simulink model "FixedWing_Dynamic_Model_SIL_PX4"  (R2022b)
settings: Solver=ode4  StartTime=0.0  StopTime=inf  FixedStep=0.004  RelTol=1e-3
model workspace (MAT data in the model file):
  sample_time = 0.004
values from neighbouring files (symbols this model uses):
  uavData = struct    [InitFixedWingParam.m]
undefined symbols (not defined in the file or in its folder): Earth, env, WGS84
libraries: aerolibactuator x5, simulink_extras x3, aerolibasang x2, aerolibatmos2 x2, shared6dof x1, aerolibtransform2 x1, aerolibconvert2 x1, aerolibanimutils x1
(part 2 of 2)

== system FixedWing_Dynamic_Model_SIL_PX4/Fixed-wing UAV Dynamics/Force and Moment Calculation/Aerodynamic Forces and Moments/Compute Body Frame Forces and Moments/Rotate FM to body frame/Rotate Moments/RB2W ==
  aoa beta : Inport
  11 : Fcn  Expr=u[3]*u[4]
  12 : Fcn  Expr=u[2]
  13 : Fcn  Expr=u[1]*u[4]
  21 : Fcn  Expr=-u[3]*u[2]
  22 : Fcn  Expr=u[4]
  23 : Fcn  Expr=-u[1]*u[2]
  31 : Fcn  Expr=-u[1]
  32 : Fcn  Expr=0
  33 : Fcn  Expr=u[3]
  Mux : Mux  Inputs=2
  Mux3 : Mux  Inputs=9
  Reshape 9x1->3x3 : Reshape  OutputDimensionality=Customize  OutputDimensions=[3,3]
  sincos : Trigonometry  Operator=sincos
  Rw2b : Outport  VectorParamsAs1DForOutWhenUnconnected=off
  wires:
  Mux/1 -> 11/1, 21/1, 31/1, 12/1, 22/1, 32/1, 13/1, 23/1, 33/1
  aoa beta/1 -> sincos/1
  sincos/2 -> Mux/2
  sincos/1 -> Mux/1
  33/1 -> Mux3/9
  23/1 -> Mux3/8
  13/1 -> Mux3/7
  32/1 -> Mux3/6
  22/1 -> Mux3/5
  12/1 -> Mux3/4
  31/1 -> Mux3/3
  21/1 -> Mux3/2
  11/1 -> Mux3/1
  Reshape 9x1->3x3/1 -> Rw2b/1
  Mux3/1 -> Reshape 9x1->3x3/1

== system FixedWing_Dynamic_Model_SIL_PX4/Fixed-wing UAV Dynamics/Force and Moment Calculation/Aerodynamic Forces and Moments/Compute Body Frame Forces and Moments/Wind frame F& M/Lateral Channel/CY ==
  beta : Inport
  dR : Inport  Port=2
  CYDr : Constant  Value=uavData.aero.CYDr
      settings: AttributesFormatString=%<Value>
  CYb : Constant  Value=uavData.aero.CYb
      settings: AttributesFormatString=%<Value>
  Product : Product  SaturateOnIntegerOverflow=on  OutDataTypeStr=Inherit: Same as first input
  Product1 : Product  SaturateOnIntegerOverflow=on  OutDataTypeStr=Inherit: Same as first input
  Sum2 : Sum  SaturateOnIntegerOverflow=on
  CY : Outport  VectorParamsAs1DForOutWhenUnconnected=off
  wires:
  Product1/1 -> Sum2/2
  dR/1 -> Product1/2
  CYDr/1 -> Product1/1
  Product/1 -> Sum2/1
  Sum2/1 -> CY/1
  beta/1 -> Product/2
  CYb/1 -> Product/1

== system FixedWing_Dynamic_Model_SIL_PX4/Fixed-wing UAV Dynamics/Force and Moment Calculation/Aerodynamic Forces and Moments/Compute Body Frame Forces and Moments/Wind frame F& M/Lateral Channel/Cl ==
  beta : Inport
  dA : Inport  Port=2
  dR : Inport  Port=3
  p,q,r : Inport  Port=4
  Airspeed : Inport  Port=5
  ClDa : Constant  Value=uavData.aero.ClDa
      settings: AttributesFormatString=%<Value>
  ClDr : Constant  Value=uavData.aero.ClDr
      settings: AttributesFormatString=%<Value>
  Clb : Constant  Value=uavData.aero.Clb
      settings: AttributesFormatString=%<Value>
  Product1 : Product  SaturateOnIntegerOverflow=on  OutDataTypeStr=Inherit: Same as first input
  Product4 : Product  SaturateOnIntegerOverflow=on  OutDataTypeStr=Inherit: Same as first input
  Product5 : Product  SaturateOnIntegerOverflow=on  OutDataTypeStr=Inherit: Same as first input
  Sum : Sum  Inputs=+++++  SaturateOnIntegerOverflow=on
  roll factors : Subsystem
  Cl : Outport  VectorParamsAs1DForOutWhenUnconnected=off
  wires:
  roll factors/1(Clp) -> Sum/4
  Product5/1 -> Sum/2  "CldA"
  Airspeed/1 -> roll factors/2(Airspeed)
  p,q,r/1 -> roll factors/1(p,q,r)
  roll factors/2(Clr) -> Sum/5
  Product1/1 -> Sum/3  "Cldr"
  Product4/1 -> Sum/1  "Clb"
  Sum/1 -> Cl/1
  dR/1 -> Product1/2
  ClDr/1 -> Product1/1
  dA/1 -> Product5/2
  ClDa/1 -> Product5/1
  beta/1 -> Product4/2
  Clb/1 -> Product4/1

== system FixedWing_Dynamic_Model_SIL_PX4/Fixed-wing UAV Dynamics/Force and Moment Calculation/Aerodynamic Forces and Moments/Compute Body Frame Forces and Moments/Wind frame F& M/Lateral Channel/Cn ==
  beta : Inport
  dA : Inport  Port=2
  Dr : Inport  Port=3
  p,q,r : Inport  Port=4
  Airspeed : Inport  Port=5
  CnDa : Constant  Value=uavData.aero.CnDa
      settings: AttributesFormatString=%<Value>
  CnDr : Constant  Value=uavData.aero.CnDr
      settings: AttributesFormatString=%<Value>
  Cnb : Constant  Value=uavData.aero.Cnb
      settings: AttributesFormatString=%<Value>
  Product1 : Product  SaturateOnIntegerOverflow=on  OutDataTypeStr=Inherit: Same as first input
  Product4 : Product  SaturateOnIntegerOverflow=on  OutDataTypeStr=Inherit: Same as first input
  Product5 : Product  SaturateOnIntegerOverflow=on  OutDataTypeStr=Inherit: Same as first input
  Sum : Sum  Inputs=+++++  SaturateOnIntegerOverflow=on
  yaw factors : Subsystem
  Cn : Outport  VectorParamsAs1DForOutWhenUnconnected=off
  wires:
  Airspeed/1 -> yaw factors/2(Airspeed)
  p,q,r/1 -> yaw factors/1(p,q,r)
  Cnb/1 -> Product4/1
  beta/1 -> Product4/2
  CnDa/1 -> Product5/1
  Product5/1 -> Sum/2
  dA/1 -> Product5/2
  CnDr/1 -> Product1/1
  Dr/1 -> Product1/2
  Sum/1 -> Cn/1
  Product1/1 -> Sum/3
  yaw factors/2(Cnr) -> Sum/5
  yaw factors/1(Cnp) -> Sum/4
  Product4/1 -> Sum/1

== system FixedWing_Dynamic_Model_SIL_PX4/Fixed-wing UAV Dynamics/Force and Moment Calculation/Aerodynamic Forces and Moments/Compute Body Frame Forces and Moments/Wind frame F& M/Longitudinal Channel/CD ==
  CL : Inport
  Apolar : Constant  Value=uavData.aero.A1
      settings: AttributesFormatString=%<Value>
  Apolar (A2) : Constant  Value=uavData.aero.Apolar
      settings: AttributesFormatString=%<Value>
  CD0 : Constant  Value=uavData.aero.CD0
      settings: AttributesFormatString=%<Value>
  Gain : Gain  Gain=-1  SaturateOnIntegerOverflow=on  OutDataTypeStr=Inherit: Same as input  ParamDataTypeStr=Inherit: Same as input
      settings: AttributesFormatString=%<Gain>
  Math Function : Math  Operator=square  SignedPower=on
  Product : Product  SaturateOnIntegerOverflow=on  OutDataTypeStr=Inherit: Same as first input
  Product1 : Product  SaturateOnIntegerOverflow=on  OutDataTypeStr=Inherit: Same as first input
  Sum1 : Sum  Inputs=+++  SaturateOnIntegerOverflow=on
  CD : Outport  VectorParamsAs1DForOutWhenUnconnected=off
  wires:
  Gain/1 -> CD/1
  Apolar (A2)/1 -> Product/1
  Math Function/1 -> Product/2
  Product1/1 -> Sum1/3
  Product/1 -> Sum1/2
  CL/1 -> Math Function/1, Product1/1
  Sum1/1 -> Gain/1
  CD0/1 -> Sum1/1
  Apolar/1 -> Product1/2

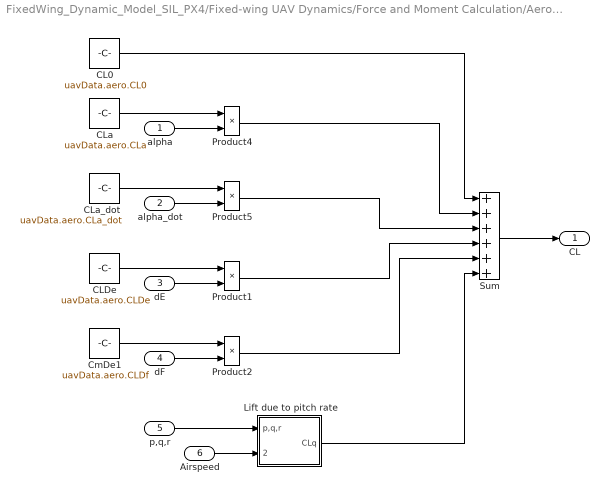
== system FixedWing_Dynamic_Model_SIL_PX4/Fixed-wing UAV Dynamics/Force and Moment Calculation/Aerodynamic Forces and Moments/Compute Body Frame Forces and Moments/Wind frame F& M/Longitudinal Channel/CL ==
  alpha : Inport
  alpha_dot : Inport  Port=2
  dE : Inport  Port=3
  dF : Inport  Port=4
  p,q,r : Inport  Port=5
  Airspeed : Inport  Port=6
  CL0 : Constant  Value=uavData.aero.CL0
      settings: AttributesFormatString=%<Value>
  CLDe : Constant  Value=uavData.aero.CLDe
      settings: AttributesFormatString=%<Value>
  CLa : Constant  Value=uavData.aero.CLa
      settings: AttributesFormatString=%<Value>
  CLa_dot : Constant  Value=uavData.aero.CLa_dot
      settings: AttributesFormatString=%<Value>
  CmDe1 : Constant  Value=uavData.aero.CLDf
      settings: AttributesFormatString=%<Value>
  Lift due to pitch rate : Subsystem
  Product{1..2,4..5} (4 alike) : Product  SaturateOnIntegerOverflow=on  OutDataTypeStr=Inherit: Same as first input
  Sum : Sum  Inputs=++++++  SaturateOnIntegerOverflow=on
  CL : Outport  VectorParamsAs1DForOutWhenUnconnected=off
  wires:
  CL0/1 -> Sum/1
  Airspeed/1 -> Lift due to pitch rate/2(Airspeed)
  p,q,r/1 -> Lift due to pitch rate/1(p,q,r)
  Lift due to pitch rate/1(CLq) -> Sum/6
  Product2/1 -> Sum/5
  Product1/1 -> Sum/4
  Product5/1 -> Sum/3
  CmDe1/1 -> Product2/1
  dF/1 -> Product2/2
  Sum/1 -> CL/1
  dE/1 -> Product1/2
  CLDe/1 -> Product1/1
  alpha_dot/1 -> Product5/2
  CLa_dot/1 -> Product5/1
  alpha/1 -> Product4/2
  CLa/1 -> Product4/1
  Product4/1 -> Sum/2

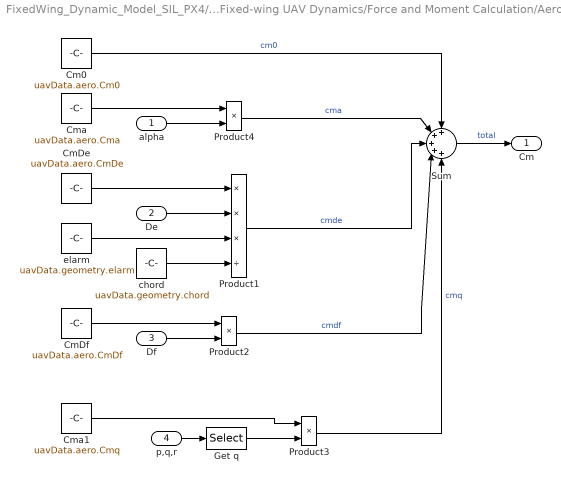
== system FixedWing_Dynamic_Model_SIL_PX4/Fixed-wing UAV Dynamics/Force and Moment Calculation/Aerodynamic Forces and Moments/Compute Body Frame Forces and Moments/Wind frame F& M/Longitudinal Channel/Cm ==
  alpha : Inport
  De : Inport  Port=2
  Df : Inport  Port=3
  p,q,r : Inport  Port=4
  Cm0 : Constant  Value=uavData.aero.Cm0
      settings: AttributesFormatString=%<Value>
  CmDe : Constant  Value=uavData.aero.CmDe
      settings: AttributesFormatString=%<Value>
  CmDf : Constant  Value=uavData.aero.CmDf
      settings: AttributesFormatString=%<Value>
  Cma : Constant  Value=uavData.aero.Cma
      settings: AttributesFormatString=%<Value>
  Cma1 : Constant  Value=uavData.aero.Cmq
      settings: AttributesFormatString=%<Value>
  Get q : Selector  InputPortWidth=3  IndexOptions=Index vector (dialog)  Indices=2  OutputSizes=[(-2)]
  Product1 : Product  Inputs=***/  SaturateOnIntegerOverflow=on  OutDataTypeStr=Inherit: Same as first input
  Product2 : Product  SaturateOnIntegerOverflow=on  OutDataTypeStr=Inherit: Same as first input
  Product3 : Product  SaturateOnIntegerOverflow=on  OutDataTypeStr=Inherit: Same as first input
  Product4 : Product  SaturateOnIntegerOverflow=on  OutDataTypeStr=Inherit: Same as first input
  Sum : Sum  Inputs=+++++  SaturateOnIntegerOverflow=on
  chord : Constant  Value=uavData.geometry.chord
      settings: AttributesFormatString=%<Value>
  elarm : Constant  Value=uavData.geometry.elarm
      settings: AttributesFormatString=%<Value>
  Cm : Outport  VectorParamsAs1DForOutWhenUnconnected=off
  wires:
  chord/1 -> Product1/4
  elarm/1 -> Product1/3
  Get q/1 -> Product3/2
  Product3/1 -> Sum/5  "cmq"
  p,q,r/1 -> Get q/1
  Cma1/1 -> Product3/1
  Product1/1 -> Sum/3  "cmde"
  Product4/1 -> Sum/2  "cma"
  Sum/1 -> Cm/1  "total"
  De/1 -> Product1/2
  CmDe/1 -> Product1/1
  alpha/1 -> Product4/2
  Cma/1 -> Product4/1
  Df/1 -> Product2/2
  CmDf/1 -> Product2/1
  Product2/1 -> Sum/4  "cmdf"
  Cm0/1 -> Sum/1  "cm0"

== system FixedWing_Dynamic_Model_SIL_PX4/Fixed-wing UAV Dynamics/Force and Moment Calculation/Aerodynamic Forces and Moments/Compute Body Frame Forces and Moments/Wind frame F& M/Lateral Channel/Cl/roll factors ==
  p,q,r : Inport
  Airspeed : Inport  Port=2
  Constant : Constant  Value=uavData.aero.Clp
      settings: AttributesFormatString=%<Value>
  Constant1 : Constant  Value=uavData.aero.Clr
      settings: AttributesFormatString=%<Value>
  Get p : Selector  InputPortWidth=3  IndexOptions=Index vector (dialog)  Indices=1  OutputSizes=[(-2)]
  Get r : Selector  InputPortWidth=3  IndexOptions=Index vector (dialog)  Indices=3  OutputSizes=[(-2)]
  Product : Product  SaturateOnIntegerOverflow=on  OutDataTypeStr=Inherit: Same as first input
  Product1 : Product  SaturateOnIntegerOverflow=on  OutDataTypeStr=Inherit: Same as first input
  roll rate fact : Subsystem
  yaw rate fact : Subsystem
  Clp : Outport  VectorParamsAs1DForOutWhenUnconnected=off
  Clr : Outport  Port=2  VectorParamsAs1DForOutWhenUnconnected=off
  wires:
  Get r/1 -> yaw rate fact/1(r)
  p,q,r/1 -> Get r/1, Get p/1
  Get p/1 -> roll rate fact/1(p)
  Airspeed/1 -> yaw rate fact/2(Airspeed), roll rate fact/2(Airspeed)
  yaw rate fact/1(Yaw Rate Fac) -> Product1/2
  Constant1/1 -> Product1/1
  roll rate fact/1(Roll Rate Fac) -> Product/2
  Constant/1 -> Product/1
  Product1/1 -> Clr/1
  Product/1 -> Clp/1

== system FixedWing_Dynamic_Model_SIL_PX4/Fixed-wing UAV Dynamics/Force and Moment Calculation/Aerodynamic Forces and Moments/Compute Body Frame Forces and Moments/Wind frame F& M/Lateral Channel/Cn/yaw factors ==
  p,q,r : Inport
  Airspeed : Inport  Port=2
  Constant : Constant  Value=uavData.aero.Cnp
      settings: AttributesFormatString=%<Value>
  Constant1 : Constant  Value=uavData.aero.Cnr
      settings: AttributesFormatString=%<Value>
  Get p : Selector  InputPortWidth=3  IndexOptions=Index vector (dialog)  Indices=1  OutputSizes=[(-2)]
  Get r : Selector  InputPortWidth=3  IndexOptions=Index vector (dialog)  Indices=3  OutputSizes=[(-2)]
  Product : Product  SaturateOnIntegerOverflow=on  OutDataTypeStr=Inherit: Same as first input
  Product1 : Product  SaturateOnIntegerOverflow=on  OutDataTypeStr=Inherit: Same as first input
  roll rate fact : Subsystem
  yaw rate fact : Subsystem
  Cnp : Outport  VectorParamsAs1DForOutWhenUnconnected=off
  Cnr : Outport  Port=2  VectorParamsAs1DForOutWhenUnconnected=off
  wires:
  Airspeed/1 -> yaw rate fact/2(Airspeed), roll rate fact/2(Airspeed)
  Get r/1 -> yaw rate fact/1(r)
  p,q,r/1 -> Get r/1, Get p/1
  Get p/1 -> roll rate fact/1(p)
  roll rate fact/1(Roll Rate Fac) -> Product/2
  Constant/1 -> Product/1
  yaw rate fact/1(Yaw Rate Fac) -> Product1/2
  Constant1/1 -> Product1/1
  Product1/1 -> Cnr/1
  Product/1 -> Cnp/1

== system FixedWing_Dynamic_Model_SIL_PX4/Fixed-wing UAV Dynamics/Force and Moment Calculation/Aerodynamic Forces and Moments/Compute Body Frame Forces and Moments/Wind frame F& M/Longitudinal Channel/CL/Lift due to pitch rate ==
  p,q,r : Inport
  Airspeed : Inport  Port=2
  Constant : Constant  Value=uavData.aero.CLq
      settings: AttributesFormatString=%<Value>
  Get q : Selector  InputPortWidth=3  IndexOptions=Index vector (dialog)  Indices=2  OutputSizes=[(-2)]
  Product : Product  SaturateOnIntegerOverflow=on  OutDataTypeStr=Inherit: Same as first input
  pitch rate factor : Subsystem
  CLq : Outport  VectorParamsAs1DForOutWhenUnconnected=off
  wires:
  Airspeed/1 -> pitch rate factor/2(Airspeed)
  Get q/1 -> pitch rate factor/1(q)
  p,q,r/1 -> Get q/1
  Product/1 -> CLq/1
  pitch rate factor/1(Pitch Rate Fac) -> Product/2
  Constant/1 -> Product/1

== system FixedWing_Dynamic_Model_SIL_PX4/Fixed-wing UAV Dynamics/Force and Moment Calculation/Aerodynamic Forces and Moments/Compute Body Frame Forces and Moments/Wind frame F& M/Lateral Channel/Cl/roll factors/roll rate fact ==
  p : Inport
  Airspeed : Inport  Port=2
  Cmq1 : Constant  Value=.5
      settings: AttributesFormatString=%<Value>
  Cmq2 : Constant  Value=uavData.geometry.span
      settings: AttributesFormatString=%<Value>
  Product : Product  Inputs=***/  SaturateOnIntegerOverflow=on  OutDataTypeStr=Inherit: Same as first input
  Saturation : Saturate  UpperLimit=inf  LowerLimit=0.1
      settings: AttributesFormatString="[%<LowerLimit>  %<UpperLimit>]"
  Roll Rate Fac : Outport  VectorParamsAs1DForOutWhenUnconnected=off
  wires:
  Saturation/1 -> Product/4
  Airspeed/1 -> Saturation/1
  Cmq2/1 -> Product/3
  Cmq1/1 -> Product/2
  p/1 -> Product/1
  Product/1 -> Roll Rate Fac/1

== system FixedWing_Dynamic_Model_SIL_PX4/Fixed-wing UAV Dynamics/Force and Moment Calculation/Aerodynamic Forces and Moments/Compute Body Frame Forces and Moments/Wind frame F& M/Lateral Channel/Cl/roll factors/yaw rate fact ==
  r : Inport
  Airspeed : Inport  Port=2
  Cmq3 : Constant  Value=.5
      settings: AttributesFormatString=%<Value>
  Cmq4 : Constant  Value=uavData.geometry.span
      settings: AttributesFormatString=%<Value>
  Product1 : Product  Inputs=***/  SaturateOnIntegerOverflow=on  OutDataTypeStr=Inherit: Same as first input
  Saturation : Saturate  UpperLimit=inf  LowerLimit=0.1
      settings: AttributesFormatString="[%<LowerLimit>  %<UpperLimit>]"
  Yaw Rate Fac : Outport  VectorParamsAs1DForOutWhenUnconnected=off
  wires:
  Product1/1 -> Yaw Rate Fac/1
  r/1 -> Product1/1
  Cmq3/1 -> Product1/2
  Cmq4/1 -> Product1/3
  Airspeed/1 -> Saturation/1
  Saturation/1 -> Product1/4

== system FixedWing_Dynamic_Model_SIL_PX4/Fixed-wing UAV Dynamics/Force and Moment Calculation/Aerodynamic Forces and Moments/Compute Body Frame Forces and Moments/Wind frame F& M/Lateral Channel/Cn/yaw factors/roll rate fact ==
  p : Inport
  Airspeed : Inport  Port=2
  Cmq1 : Constant  Value=.5
      settings: AttributesFormatString=%<Value>
  Cmq2 : Constant  Value=uavData.geometry.span
      settings: AttributesFormatString=%<Value>
  Product : Product  Inputs=***/  SaturateOnIntegerOverflow=on  OutDataTypeStr=Inherit: Same as first input
  Saturation : Saturate  UpperLimit=inf  LowerLimit=0.1
      settings: AttributesFormatString="[%<LowerLimit>  %<UpperLimit>]"
  Roll Rate Fac : Outport  VectorParamsAs1DForOutWhenUnconnected=off
  wires:
  Saturation/1 -> Product/4
  Airspeed/1 -> Saturation/1
  Cmq2/1 -> Product/3
  Cmq1/1 -> Product/2
  p/1 -> Product/1
  Product/1 -> Roll Rate Fac/1

== system FixedWing_Dynamic_Model_SIL_PX4/Fixed-wing UAV Dynamics/Force and Moment Calculation/Aerodynamic Forces and Moments/Compute Body Frame Forces and Moments/Wind frame F& M/Lateral Channel/Cn/yaw factors/yaw rate fact ==
  r : Inport
  Airspeed : Inport  Port=2
  Cmq3 : Constant  Value=.5
      settings: AttributesFormatString=%<Value>
  Cmq4 : Constant  Value=uavData.geometry.span
      settings: AttributesFormatString=%<Value>
  Product1 : Product  Inputs=***/  SaturateOnIntegerOverflow=on  OutDataTypeStr=Inherit: Same as first input
  Saturation : Saturate  UpperLimit=inf  LowerLimit=0.1
      settings: AttributesFormatString="[%<LowerLimit>  %<UpperLimit>]"
  Yaw Rate Fac : Outport  VectorParamsAs1DForOutWhenUnconnected=off
  wires:
  Product1/1 -> Yaw Rate Fac/1
  r/1 -> Product1/1
  Cmq3/1 -> Product1/2
  Cmq4/1 -> Product1/3
  Airspeed/1 -> Saturation/1
  Saturation/1 -> Product1/4

== system FixedWing_Dynamic_Model_SIL_PX4/Fixed-wing UAV Dynamics/Force and Moment Calculation/Aerodynamic Forces and Moments/Compute Body Frame Forces and Moments/Wind frame F& M/Longitudinal Channel/CL/Lift due to pitch rate/pitch rate factor ==
  q : Inport
  Airspeed : Inport  Port=2
  Cmq2 : Constant  Value=uavData.geometry.chord
      settings: AttributesFormatString=%<Value>
  Product : Product  Inputs=**/  SaturateOnIntegerOverflow=on  OutDataTypeStr=Inherit: Same as first input
  Saturation : Saturate  UpperLimit=inf  LowerLimit=0.1
      settings: AttributesFormatString="[%<LowerLimit>  %<UpperLimit>]"
  Pitch Rate Fac : Outport  VectorParamsAs1DForOutWhenUnconnected=off
  wires:
  Saturation/1 -> Product/3
  Cmq2/1 -> Product/2
  Airspeed/1 -> Saturation/1
  q/1 -> Product/1
  Product/1 -> Pitch Rate Fac/1

== matlab function FixedWing_Dynamic_Model_SIL_PX4/Radio/PWM Mapping ==
  data: analog input; pwm1 output; pwm2 output; pwm3 output; pwm4 output; pwm5 output; buttons input; pwm6 output; pwm7 output; pwm8 output; pwm9 output
function [pwm1,pwm2,pwm3,pwm4,pwm5,pwm6,pwm7,pwm8,pwm9] = pmw_mapping(analog,buttons)

analog=round(analog*100)/100;
pwm1=(analog(1)+1)*500+1000;
pwm2=(analog(2)+1)*500+1000;
pwm3=analog(3)*1000+1000;
pwm4=(analog(4)+1)*500+1000;
pwm5=1000;
pwm6=1000;
pwm7=1000;
pwm8=1000;
pwm9=1000;

if buttons==1
    pwm5=2000;
elseif buttons==16
    pwm6=2000;
elseif buttons==32
    pwm7=2000;
elseif buttons==64
    pwm8=2000;
elseif buttons==128
    pwm9=2000;
end

== matlab function FixedWing_Dynamic_Model_SIL_PX4/Pixhawk SITL/GNSS/MATLAB Function1 ==
  data: course input; course output
function course = wrapToMaxCourse(course)

    isPositive = (course > 0);
    course = mod(course, 360);
    course((course == 0) & isPositive) = 360;

end

== matlab function FixedWing_Dynamic_Model_SIL_PX4/Pixhawk SITL/Ground truth/Euler angles and Euler angle rates ==
  data: phitehtapsi output; phitehtapsi input; phithetapsi_dot output; pqr input
function [phitehtapsi,phithetapsi_dot] = euler_angle_rates(phitehtapsi,pqr)
    
    phi=phitehtapsi(1);
    theta=phitehtapsi(2);

    sphi=sin(phi);
    cphi=cos(phi);
    stheta=sin(theta);
    ctheta=cos(theta);

    phithetapsi_dot=[1,sphi*stheta/ctheta,cphi*stheta/ctheta;
        0,cphi,-sphi;
        0,sphi/ctheta,cphi/ctheta]*pqr;
